simulink model "Simulatie_integral"  (R2018b)
settings: Solver=FixedStepAuto  StartTime=0.0  StopTime=inf  FixedStep=1e-5  RelTol=1e-3
values from neighbouring files (symbols this model uses):
  A = [-(bm*(n^2) + bg)/(Jm*(n^2) + Jg) Kt*n/(Jm*(n^2) + Jg) ... (first row only)    [DC_motor_geared_integral_discrete_sysid23.m]    (also in DC_motor_geared_lqr_discrete_sysid23.m; finalScript.m; finalScriptV2.m; precompensatorVSintegrator.m)
  B = [0 ... (first row only)    [DC_motor_geared_integral_discrete_sysid23.m]    (also in DC_motor_geared_lqr_discrete_sysid23.m; finalScript.m; finalScriptV2.m; precompensatorVSintegrator.m)
  C = [1 0]    [DC_motor_geared_integral_discrete_sysid23.m]    (also in DC_motor_geared_lqr_discrete_sysid23.m = eye(2); finalScript.m; finalScriptV2.m; precompensatorVSintegrator.m = eye(2))
  D = [0]    [DC_motor_geared_integral_discrete_sysid23.m]    (also in DC_motor_geared_lqr_discrete_sysid23.m = [0;0]; finalScript.m; finalScriptV2.m; precompensatorVSintegrator.m)
  Kdi = dlqr(Ad,Bd,Q,R)    [DC_motor_geared_integral_discrete_sysid23.m]    (also in finalScript.m; finalScriptV2.m)
  n = 16.5    [DC_motor_geared_integral_discrete_sysid23.m]    (also in DC_motor_geared_lqr_discrete_sysid23.m; finalScript.m; finalScriptV2.m)
  Tsc = 1/20000    (= 5e-05)    [DC_motor_geared_integral_discrete_sysid23.m]    (also in DC_motor_geared_lqr_discrete_sysid23.m = 1e-05; finalScript.m; finalScriptV2.m = 0.001)
undefined symbols (not defined in the file or in its folder): Add, Bdd, DiscIntNeverNeededParam, sigbuilder_block
libraries: dspswit3 x22, powerlib_meascontrol x17, simulink x11, dspsigops x4, peLuenbergerObserver x2, peGeneralControl x1
settings Model: Creator=BooJC  LastModifiedBy=Roberto
settings SolverCC: AlgebraicLoopSolver=LineSearch
settings DataIOCC: ExternalInput=v_motor_ts
settings DebuggingCC: LibraryContextMissingDiagnostic=none
settings SFSimCC: SimUseLocalCustomCode=off
settings RTWCC: RTWUseLocalCustomCode=off

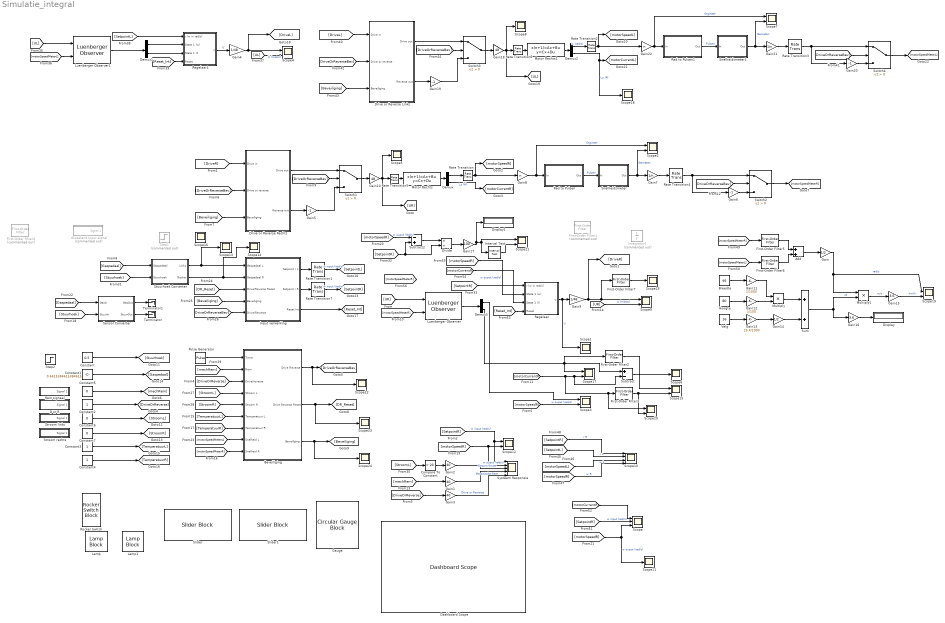
== system Simulatie_integral ==
  Add : Sum
  Beveiliging : Subsystem
  Breedte : Constant  Value=95
  Compare To Constant : simulink/Logic and Bit Operations/Compare To Constant  relop=>  const=20  OutDataTypeStr=boolean
  Constant : Constant  Value=0.5  SampleTime=1/1000
  Constant1 : Constant  Value=0.6615384615384615
  Constant2 : Constant
  Constant3 : Constant
  Constant4 : Constant
  Constant5 : Constant  Value=0
  Constant6 : Constant  Value=0
  Constant7 : Constant  Value=0
  D or R : Subsystem  Tag=STV Subsys  LoadFcn=sigbuilder_block('load');  StartFcn=sigbuilder_block('start');  StopFcn=sigbuilder_block('stop');  ClipboardFcn=sigbuilder_block('clipboard');  mask(Sigbuilder block){tuvar=[0:10]}
      mask help: Simulink:masks:SigbuilderBlock_MD
      mask init:
      | if ~strcmp(get_param(bdroot(gcbh),'SimulationStatus'),'stopped') tuvar = sigbuilder_block('maskInit'); end
      settings: CopyFcn=sigbuilder_block('copy');  DeleteFcn=sigbuilder_block('delete');  ModelCloseFcn=sigbuilder_block('modelClose');  PreSaveFcn=sigbuilder_block('preSave');  PauseFcn=sigbuilder_block('pause');  ContinueFcn=sigbuilder_block('continue');  NameChangeFcn=sigbuilder_block('namechange');  OpenFcn=sigbuilder_block('open',[437.6 153 550.4 359.25 ]);  CloseFcn=sigbuilder_block('close');
      mask Display: plot(0, 0, 100, 100,[2, 2, 32, 32, 2], [68, 8, 8, 68, 68],[32, 2], [38, 38], [32, 19, 2],[53, 60, 44], [32, 17, 17, 2],[16, 16, 31, 31]);txt = getActiveGroup(gcbh);text(2, 100, txt,'verticalAlignment', 'top');
  Dashboard Scope : DashboardScope  WebBlockId=1704  Ymin=-20  Ymax=20
  Demux{,1..3} (4 alike) : Demux  Outputs=2
  Display : Display
  Display1 : Display
  Divide : Product  Inputs=*/
  Drive or Reverse Links : Subsystem
  Drive or Reverse Rechts : Subsystem
  First-Order Filter1 : powerlib_meascontrol/Filters/First-Order Filter  Commented=on  FilterType=Lowpass  Tc=10e-2  Ts=Tsc  Initialize=on  Vac_Init=[0, 0, 50]  Vdc_Init=0  PlotResponse=off  FreqRange="[0,  200,  1]"
      settings: SourceProductName=Simscape Power Systems
  First-Order Filter{2..3,5..7} (5 alike) : powerlib_meascontrol/Filters/First-Order Filter  FilterType=Lowpass  Tc=10e-3  Ts=Tsc  Initialize=on  Vac_Init=[0, 0, 50]  Vdc_Init=0  PlotResponse=off  FreqRange="[0,  200,  1]"
      settings: SourceProductName=Simscape Power Systems
  First-Order Filter4 : powerlib_meascontrol/Filters/First-Order Filter  Commented=on  FilterType=Lowpass  Tc=10e-1  Ts=Tsc  Initialize=on  Vac_Init=[0, 0, 50]  Vdc_Init=0  PlotResponse=off  FreqRange="[0,  200,  1]"
      settings: SourceProductName=Simscape Power Systems
  Gain : Gain  Gain=1/2
  Gain1 : Gain  Gain=40
  Gain10 : Gain  Gain=48
  Gain11 : Gain  Gain=1/1000
  Gain12 : Gain  Gain=1/100
  Gain13 : Gain  Gain=25.4/1000
  Gain14 : Gain  Gain=1/2
  Gain15 : Gain  Gain=3.6
  Gain16 : Gain  Gain=3.6
  Gain17 : Gain  Gain=100
  Gain18 : Gain  Gain=48
  Gain{5..6,19..20} (4 alike) : Gain  Gain=-1
  Gain2 : Gain  Gain=40
  Gain21 : Gain  Gain=1/n
  Gain22 : Gain  Gain=n
  Gain3 : Gain  Gain=40
  Gain4 : Gain  Gain=1/48
  Gain7 : Gain  Gain=1/n
  Gain8 : Gain  Gain=n
  Gain9 : Gain  Gain=1/48
  Gauge : CircularGaugeBlock  WebBlockId=1560  ScaleMin=-50  ScaleMax=50
  Hoogte : Constant  Value=80
  Input verwerking : Subsystem
  Integrator1 : Integrator  Commented=on
  Interval Test : simulink/Logic and Bit Operations/Interval Test  IntervalClosedRight=on  uplimit=2  IntervalClosedLeft=on  lowlimit=-2  OutDataTypeStr=boolean
  Lamp : LampBlock  WebBlockId=1564
  Lamp1 : LampBlock  WebBlockId=1565
  Luenberger Observer : peLuenbergerObserver/Luenberger Observer  StateSpaceType=Discrete-time  Ad=Add  Bd=Bdd  Cd=[1 0]  Dd=0  A=A  B=B  C=C  D=D  ObserverDesign=Observer gain  Ld=L  DesiredEigenvalues=eigenVal  x0=[0 0]  Tsd=0.1  Ts=Tsc
  Luenberger Observer1 : peLuenbergerObserver/Luenberger Observer  StateSpaceType=Discrete-time  Ad=Add  Bd=Bdd  Cd=[1 0]  Dd=0  A=A  B=B  C=C  D=D  ObserverDesign=Observer gain  Ld=L  DesiredEigenvalues=eigenVal  x0=[0 0]  Tsd=0.1  Ts=Tsc
  Motor Rechts : DiscreteStateSpace  A=Add  B=Bdd  C=eye(2)  D=[0; 0]  SampleTime=Tsc
  Motor Rechts1 : DiscreteStateSpace  A=Add  B=Bdd  C=eye(2)  D=[0; 0]  SampleTime=Tsc
  Multiply : Product
  Multiply1 : Product
  Pulse Generator : DiscretePulseGenerator  SampleTime=1/2000
  Rad to Pulsen : Subsystem
  Rad to Pulsen1 : Subsystem
  Rate Transition : RateTransition  OutPortSampleTime=1/100000
  Rate Transition{1,3..7} (6 alike) : RateTransition  OutPortSampleTime=Tsc
  Rate Transition2 : RateTransition  OutPortSampleTime=1/100000
  Regelaar : Subsystem
  Regelaar1 : Subsystem
  Rem signaal : Subsystem  Tag=STV Subsys  LoadFcn=sigbuilder_block('load');  StartFcn=sigbuilder_block('start');  StopFcn=sigbuilder_block('stop');  ClipboardFcn=sigbuilder_block('clipboard');  mask(Sigbuilder block){tuvar=[0:10]}
      mask help: Simulink:masks:SigbuilderBlock_MD
      mask init:
      | if ~strcmp(get_param(bdroot(gcbh),'SimulationStatus'),'stopped') tuvar = sigbuilder_block('maskInit'); end
      settings: CopyFcn=sigbuilder_block('copy');  DeleteFcn=sigbuilder_block('delete');  ModelCloseFcn=sigbuilder_block('modelClose');  PreSaveFcn=sigbuilder_block('preSave');  PauseFcn=sigbuilder_block('pause');  ContinueFcn=sigbuilder_block('continue');  NameChangeFcn=sigbuilder_block('namechange');  OpenFcn=sigbuilder_block('open',[437.6 153 550.4 359.25 ]);  CloseFcn=sigbuilder_block('close');
      mask Display: plot(0, 0, 100, 100,[2, 2, 32, 32, 2], [68, 8, 8, 68, 68],[32, 2], [38, 38], [32, 19, 2],[53, 60, 44], [32, 17, 17, 2],[16, 16, 31, 31]);txt = getActiveGroup(gcbh);text(2, 100, txt,'verticalAlignment', 'top');
  Rocker Switch : RockerSwitchBlock  WebBlockId=1563
      settings: Values={{'Off', 'On'}, [0 1]}
  Scope : Scope  NumInputPorts=3
  Scope{1,5..6,8,11,13..14,16,18,22..25} (13 alike) : Scope
  Scope10 : Scope  NumInputPorts=4
  Scope{2..4,7,9,12,15,17,19..21} (11 alike) : Scope  NumInputPorts=2
  Sensor Converter : Subsystem
  Slider : SliderBlock  WebBlockId=1558  ScaleMax=1
  Slider1 : SliderBlock  WebBlockId=1559  ScaleMax=1
  Snelheidsmeter : Subsystem
  Snelheidsmeter1 : Subsystem
  Step1 : Step  Commented=on  After=3.3  SampleTime=1/100000
  Step2 : Step  Time=0.1  SampleTime=0
  Stroom links : Subsystem  Tag=STV Subsys  LoadFcn=sigbuilder_block('load');  StartFcn=sigbuilder_block('start');  StopFcn=sigbuilder_block('stop');  ClipboardFcn=sigbuilder_block('clipboard');  mask(Sigbuilder block){tuvar=[0:10]}
      mask help: Simulink:masks:SigbuilderBlock_MD
      mask init:
      | if ~strcmp(get_param(bdroot(gcbh),'SimulationStatus'),'stopped') tuvar = sigbuilder_block('maskInit'); end
      settings: CopyFcn=sigbuilder_block('copy');  DeleteFcn=sigbuilder_block('delete');  ModelCloseFcn=sigbuilder_block('modelClose');  PreSaveFcn=sigbuilder_block('preSave');  PauseFcn=sigbuilder_block('pause');  ContinueFcn=sigbuilder_block('continue');  NameChangeFcn=sigbuilder_block('namechange');  OpenFcn=sigbuilder_block('open',[437.6 153 550.4 359.25 ]);  CloseFcn=sigbuilder_block('close');
      mask Display: plot(0, 0, 100, 100,[2, 2, 32, 32, 2], [68, 8, 8, 68, 68],[32, 2], [38, 38], [32, 19, 2],[53, 60, 44], [32, 17, 17, 2],[16, 16, 31, 31]);txt = getActiveGroup(gcbh);text(2, 100, txt,'verticalAlignment', 'top');
  Stroom rechts : Subsystem  Tag=STV Subsys  LoadFcn=sigbuilder_block('load');  StartFcn=sigbuilder_block('start');  StopFcn=sigbuilder_block('stop');  ClipboardFcn=sigbuilder_block('clipboard');  mask(Sigbuilder block){tuvar=[0:10]}
      mask help: Simulink:masks:SigbuilderBlock_MD
      mask init:
      | if ~strcmp(get_param(bdroot(gcbh),'SimulationStatus'),'stopped') tuvar = sigbuilder_block('maskInit'); end
      settings: CopyFcn=sigbuilder_block('copy');  DeleteFcn=sigbuilder_block('delete');  ModelCloseFcn=sigbuilder_block('modelClose');  PreSaveFcn=sigbuilder_block('preSave');  PauseFcn=sigbuilder_block('pause');  ContinueFcn=sigbuilder_block('continue');  NameChangeFcn=sigbuilder_block('namechange');  OpenFcn=sigbuilder_block('open',[437.6 153 550.4 359.25 ]);  CloseFcn=sigbuilder_block('close');
      mask Display: plot(0, 0, 100, 100,[2, 2, 32, 32, 2], [68, 8, 8, 68, 68],[32, 2], [38, 38], [32, 19, 2],[53, 60, 44], [32, 17, 17, 2],[16, 16, 31, 31]);txt = getActiveGroup(gcbh);text(2, 100, txt,'verticalAlignment', 'top');
  Stuurhoek Converter : Subsystem
  Subtract : Sum  Inputs=+-
  Subtract2 : Sum  Inputs=-+
  Sum : Sum
  Switch{1..4} (4 alike) : Switch  Criteria=u2 > Threshold
  Systeem Responsie : Scope  NumInputPorts=5
  Terminator : Terminator
  Terminator1 : Terminator
  Velg : Constant  Value=16
  Wisselend Input signal : Subsystem  Tag=STV Subsys  Commented=on  LoadFcn=sigbuilder_block('load');  StartFcn=sigbuilder_block('start');  StopFcn=sigbuilder_block('stop');  ClipboardFcn=sigbuilder_block('clipboard');  mask(Sigbuilder block){tuvar=[0:10]}
      mask help: Simulink:masks:SigbuilderBlock_MD
      mask init:
      | if ~strcmp(get_param(bdroot(gcbh),'SimulationStatus'),'stopped') tuvar = sigbuilder_block('maskInit'); end
      settings: CopyFcn=sigbuilder_block('copy');  DeleteFcn=sigbuilder_block('delete');  ModelCloseFcn=sigbuilder_block('modelClose');  PreSaveFcn=sigbuilder_block('preSave');  PauseFcn=sigbuilder_block('pause');  ContinueFcn=sigbuilder_block('continue');  NameChangeFcn=sigbuilder_block('namechange');  OpenFcn=sigbuilder_block('open',[437.6 153 550.4 359.25 ]);  CloseFcn=sigbuilder_block('close');
      mask Display: plot(0, 0, 100, 100,[2, 2, 32, 32, 2], [68, 8, 8, 68, 68],[32, 2], [38, 38], [32, 19, 2],[53, 60, 44], [32, 17, 17, 2],[16, 16, 31, 31]);txt = getActiveGroup(gcbh);text(2, 100, txt,'verticalAlignment', 'top');
  wires:
  Rate Transition1/1 -> [SetpointL]  "w input (rad/s)"
  Demux/2 -> [motorCurrentR]  "I_s (A)"
  Constant5/1 -> [mechRem]
  [DriveR] -> Drive or Reverse Rechts/1(Drive in)
  [DriveOrReverseBev] -> Drive or Reverse Rechts/2(Drive or reverse)
  Demux3/2 -> First-Order Filter2/1, Scope17/1, Subtract/1
  [motorCurrentR] -> Scope20/1, First-Order Filter3/1, Subtract/2, Scope17/2
  [motorSpeedR] -> Scope3/2  "w ouput (rad/s)"
  Demux3/1 -> Scope3/1
  Rad to Pulsen/1(Out) -> Snelheidsmeter/1(In)  "Pulsen"
  [motorSpeedMeterR] -> Luenberger Observer/2
  Snelheidsmeter/1(Out) -> Gain7/1, Scope2/2  "Gemeten"
  Gain8/1 -> Rad to Pulsen/1(In), Scope2/1  "Orgineel"
  Gain7/1 -> Rate Transition4/1
  Gain10/1 -> Rate Transition5/1, Scope5/1, [UR]
  [UR] -> Luenberger Observer/1
  Subtract/1 -> Scope6/1
  Rate Transition/1 -> [motorSpeedR], Gain8/1
  Regelaar/1(u) -> Scope1/1, Gain9/1  "U"
  Rate Transition5/1 -> Motor Rechts/1
  [UR] -> Scope9/2  "U (motor)"
  Pulse Generator/1 -> Beveiliging/1(Timer)
  Drive or Reverse Rechts/1(Drive out) -> Switch1/1
  Drive or Reverse Rechts/2(Reverse out) -> Gain5/1
  Switch1/1 -> Gain10/1
  [DriveOrReverseBev] -> Switch1/2
  Gain5/1 -> Switch1/3
  Gain6/1 -> Switch2/3
  Rate Transition4/1 -> Gain6/1, Switch2/1
  Switch2/1 -> [motorSpeedMeterR]
  First-Order Filter2/1 -> Scope15/1
  First-Order Filter3/1 -> Scope20/2, Scope15/2
  Gain9/1 -> [DriveR], First-Order Filter7/1, Scope9/1
  [Gaspedaal] -> Stuurhoek Converter/1("Gaspedaal ")
  [Beveiliging] -> Drive or Reverse Rechts/3(Beveiliging)
  Hoogte/1 -> Gain12/1
  Gain11/1 -> Multiply/1
  Gain13/1 -> Gain14/1
  Breedte/1 -> Gain11/1
  Gain14/1 -> Sum/2
  Multiply/1 -> Sum/1
  Gain12/1 -> Multiply/2
  Velg/1 -> Gain13/1
  Gain/1 -> Multiply1/1, Scope19/1  "rad/s"
  Sum/1 -> Gain16/1, Multiply1/2  "r0"
  Multiply1/1 -> Gain15/1  "m/s"
  Gain15/1 -> Scope19/2  "km/h"
  Gain16/1 -> Display/1
  Input verwerking/1(Setpoint r L) -> Rate Transition1/1
  [Stuurhoek] -> Stuurhoek Converter/2(Stuurhoek)
  [motorSpeedR] -> Subtract2/1  "w ouput (rad/s)"
  Subtract2/1 -> Divide/1
  Gain17/1 -> Display1/1, Interval Test/1, Scope21/1
  Divide/1 -> Gain17/1
  [motorSpeedMeterL] -> Beveiliging/8(Snelheid L)
  [motorSpeedMeterR] -> Beveiliging/9(Snelheid R)
  [StroomL] -> Beveiliging/4(Stroom L)
  [DR_Reset] -> Input verwerking/3(Drive/Reverse Reset)
  Beveiliging/3(Beveiliging) -> Scope24/1, [Beveiliging]
  [Beveiliging] -> Input verwerking/4(Beveiliging)
  [DriveOrReverse] -> Beveiliging/3(Drive/reverse)
  Beveiliging/1("Drive Reverse ") -> Scope22/1, [DriveOrReverseBev]
  [DriveOrReverseBev] -> Input verwerking/5(Drive/Reverse)
  [DriveOrReverseBev] -> Switch2/2
  Gain3/1 -> Systeem Responsie/5  "Drive or Reverse"
  [mechRem] -> Gain1/1
  Compare To Constant/1 -> Gain2/1
  Gain2/1 -> Systeem Responsie/3  "Stroom limiet"
  [DriveOrReverse] -> Gain3/1
  [motorSpeedR] -> Scope12/2, Systeem Responsie/2  "w ouput (rad/s)"
  [SetpointR] -> Scope12/1, Systeem Responsie/1  "w input (rad/s)"
  Gain1/1 -> Systeem Responsie/4  "Mecanische Rem"
  [StroomL] -> Compare To Constant/1
  Luenberger Observer/1 -> Demux3/1
  Constant2/1 -> [DriveOrReverse]
  Constant6/1 -> [StroomL]
  Constant7/1 -> [StroomR]
  Constant/1 -> [Stuurhoek]
  Constant1/1 -> [Gaspedaal]
  Constant3/1 -> [TemperatuurL]
  Constant4/1 -> [TemperatuurR]
  [TemperatuurL] -> Beveiliging/6(Temperatuur L)
  [TemperatuurR] -> Beveiliging/7(Temperatuur R)
  [StroomR] -> Beveiliging/5(Stroom R)
  [mechRem] -> Beveiliging/2(Rem)
  [Stuurhoek] -> Sensor Converter/2(StuurIn)
  [Gaspedaal] -> Sensor Converter/1(GasIn)
  Sensor Converter/2(StuurOut) -> Terminator/1
  Sensor Converter/1(GasOut) -> Terminator1/1
  Input verwerking/3(Reset Int) -> [Reset_Int]
  [SetpointR] -> Divide/2, Subtract2/2
  [SetpointR] -> Regelaar/1(r (w in rad/s))
  [Reset_Int] -> Regelaar/4(Reset)
  [UL] -> Scope4/2  "U (motor)"
  [motorSpeedMeterL] -> Luenberger Observer1/2
  [UL] -> Luenberger Observer1/1
  Gain4/1 -> [DriveL], Scope4/1
  Regelaar1/1(u) -> Gain4/1  "U"
  Luenberger Observer1/1 -> Demux1/1
  [Reset_Int] -> Regelaar1/4(Reset)
  [SetpointL] -> Regelaar1/1(r (w in rad/s))
  Drive or Reverse Links/2(Reverse out) -> Gain19/1
  Switch3/1 -> Gain18/1
  [DriveL] -> Drive or Reverse Links/1(Drive in)
  Switch4/1 -> [motorSpeedMeterL]
  Gain20/1 -> Switch4/3
  Gain22/1 -> Rad to Pulsen1/1(In), Scope7/1  "Orgineel"
  Drive or Reverse Links/1(Drive out) -> Switch3/1
  [Beveiliging] -> Drive or Reverse Links/3(Beveiliging)
  Gain19/1 -> Switch3/3
  Demux2/1 -> Rate Transition2/1  "w (rad/s)"
  Gain18/1 -> Rate Transition6/1, Scope8/1, [UL]
  Rate Transition2/1 -> [motorSpeedL], Gain22/1
  Rate Transition3/1 -> Gain20/1, Switch4/1
  Motor Rechts1/1 -> Demux2/1
  Gain21/1 -> Rate Transition3/1
  Rate Transition6/1 -> Motor Rechts1/1
  Snelheidsmeter1/1(Out) -> Gain21/1, Scope7/2  "Gemeten"
  [DriveOrReverseBev] -> Drive or Reverse Links/2(Drive or reverse)
  [DriveOrReverseBev] -> Switch3/2
  Demux2/2 -> Scope18/1, [motorCurrentL]  "I_s (A)"
  Rad to Pulsen1/1(Out) -> Snelheidsmeter1/1(In)  "Pulsen"
  [DriveOrReverseBev] -> Switch4/2
  [SetpointL] -> Scope10/2  "r L"
  [motorSpeedL] -> Scope10/3  "w L"
  [motorSpeedR] -> Scope10/4  "w R"
  Stuurhoek Converter/1(Links) -> Scope13/1, Input verwerking/1(Gaspedaal L)
  Stuurhoek Converter/2(Rechts) -> Scope14/1, Input verwerking/2(Gaspedaal R)
  Rate Transition7/1 -> [SetpointR]  "w input (rad/s)"
  Input verwerking/2(Setpoint r R) -> Rate Transition7/1
  [SetpointR] -> Scope10/1  "r R"
  [motorSpeedMeterR] -> First-Order Filter5/1
  First-Order Filter5/1 -> Add/1
  First-Order Filter6/1 -> Add/2
  [motorSpeedMeterL] -> First-Order Filter6/1
  Add/1 -> Gain/1
  [motorSpeedR] -> Scope11/1, Scope/3  "w ouput (rad/s)"
  [SetpointR] -> Scope/2  "w input (rad/s)"
  [motorCurrentR] -> Scope/1
  Interval Test/1 -> Scope21/2
  Beveiliging/2(Drive Reverse Reset) -> Scope23/1, [DR_Reset]
  Motor Rechts/1 -> Demux/1
  Demux/1 -> Rate Transition/1
  Demux1/1 -> Regelaar1/2(State 1 (w))
  Demux1/2 -> Regelaar1/3(State 1 (I))
  First-Order Filter7/1 -> Scope25/1
  [motorSpeedR] -> Regelaar/2(State 1 (w))  "w ouput (rad/s)"
  [motorCurrentR] -> Regelaar/3(State 1 (I))

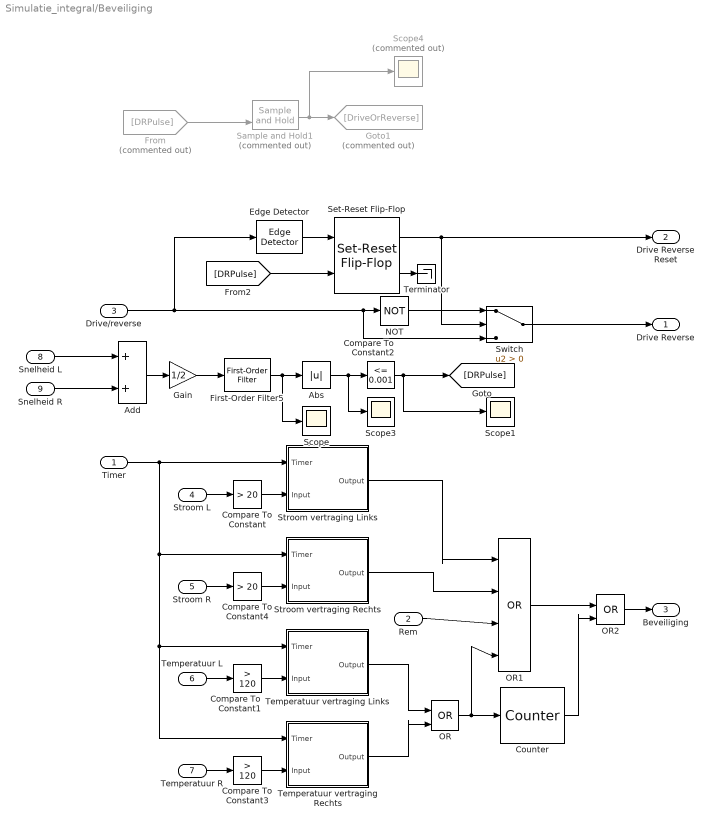
== system Simulatie_integral/Beveiliging ==
  Timer : Inport
  Rem : Inport  Port=2
  Drive/reverse : Inport  Port=3
  Stroom L : Inport  Port=4
  Stroom R : Inport  Port=5
  Temperatuur L : Inport  Port=6
  Temperatuur R : Inport  Port=7
  Snelheid L : Inport  Port=8
  Snelheid R : Inport  Port=9
  Abs : Abs
  Add : Sum
  Compare To Constant : simulink/Logic and Bit Operations/Compare To Constant  relop=>  const=20  OutDataTypeStr=boolean
  Compare To Constant1 : simulink/Logic and Bit Operations/Compare To Constant  relop=>  const=120  OutDataTypeStr=boolean
  Compare To Constant2 : simulink/Logic and Bit Operations/Compare To Constant  relop=<=  const=0.001  OutDataTypeStr=boolean
  Compare To Constant3 : simulink/Logic and Bit Operations/Compare To Constant  relop=>  const=120  OutDataTypeStr=boolean
  Compare To Constant4 : simulink/Logic and Bit Operations/Compare To Constant  relop=>  const=20  OutDataTypeStr=boolean
  Counter : dspswit3/Counter  Direction=Up  CountEvent=Rising edge  CounterSize=32 bits  MaxCount=255  InitialCount=0  Output=Hit  HitValue=3  ResetInput=off  SamplesPerFrame=1  Ts=1  CntDtype=double  HitDtype=Logical
  Edge Detector : powerlib_meascontrol/Logic/Edge Detector  model=Either  ic=0  Ts=-1
      settings: SourceProductName=Simscape Power Systems  SourceProductBaseCode=PS
  First-Order Filter5 : powerlib_meascontrol/Filters/First-Order Filter  FilterType=Lowpass  Tc=10e-3  Ts=Tsc  Initialize=on  Vac_Init=[0, 0, 50]  Vdc_Init=0  PlotResponse=off  FreqRange="[0,  200,  1]"
      settings: SourceProductName=Simscape Power Systems
  From : From  Commented=on  GotoTag=DRPulse
  Gain : Gain  Gain=1/2
  Goto1 : Goto  Commented=on  GotoTag=DriveOrReverse
  NOT : Logic  Operator=NOT  IconShape=distinctive  AllPortsSameDT=off  OutDataTypeStr=boolean
  OR : Logic  Operator=OR  IconShape=distinctive  AllPortsSameDT=off  OutDataTypeStr=boolean
  OR1 : Logic  Operator=OR  Inputs=4  IconShape=distinctive  AllPortsSameDT=off  OutDataTypeStr=boolean
  OR2 : Logic  Operator=OR  IconShape=distinctive  AllPortsSameDT=off  OutDataTypeStr=boolean
  Sample and Hold1 : powerlib_meascontrol/Additional Components/Sample and Hold  Commented=on  ic=0  Ts=0
      settings: SourceProductName=Simscape Power Systems  SourceProductBaseCode=PS
  Scope : Scope
  Scope1 : Scope
  Scope3 : Scope
  Scope4 : Scope  Commented=on
  Set-Reset Flip-Flop : peGeneralControl/Set-Reset Flip-Flop  LabelModeActiveChoice=Discrete  UndefState=Set  Q0=0  Ts=-1
  Stroom vertraging Links : Subsystem
  Stroom vertraging Rechts : Subsystem
  Switch : Switch  Criteria=u2 > Threshold
  Temperatuur vertraging Links : Subsystem
  "Temperatuur vertraging Rechts " : Subsystem
  Terminator : Terminator
  "Drive Reverse " : Outport
  Drive Reverse Reset : Outport  Port=2
  Beveiliging : Outport  Port=3
  wires:
  Compare To Constant/1 -> Stroom vertraging Links/2(Input)
  Stroom L/1 -> Compare To Constant/1
  Compare To Constant1/1 -> Temperatuur vertraging Links/2(Input)
  Temperatuur L/1 -> Compare To Constant1/1
  Edge Detector/1 -> Set-Reset Flip-Flop/1
  Set-Reset Flip-Flop/1 -> Switch/2, Drive Reverse Reset/1
  Sample and Hold1/1 -> Scope4/1, Goto1/1
  Abs/1 -> Scope3/1, Compare To Constant2/1
  Compare To Constant2/1 -> [DRPulse], Scope1/1
  [DRPulse] -> Set-Reset Flip-Flop/2
  Drive/reverse/1 -> Edge Detector/1, Switch/3, NOT/1
  From/1 -> Sample and Hold1/2
  Snelheid L/1 -> Add/1
  Snelheid R/1 -> Add/2
  Add/1 -> Gain/1
  Gain/1 -> First-Order Filter5/1
  Compare To Constant3/1 -> "Temperatuur vertraging Rechts "/2(Input)
  Timer/1 -> Stroom vertraging Links/1(Timer), Stroom vertraging Rechts/1(Timer), "Temperatuur vertraging Rechts "/1(Timer), Temperatuur vertraging Links/1(Timer)
  Compare To Constant4/1 -> Stroom vertraging Rechts/2(Input)
  Stroom R/1 -> Compare To Constant4/1
  Rem/1 -> OR1/3
  Stroom vertraging Links/1(Output) -> OR1/1
  Stroom vertraging Rechts/1(Output) -> OR1/2
  Switch/1 -> "Drive Reverse "/1
  NOT/1 -> Switch/1
  OR/1 -> OR1/4, Counter/1
  Temperatuur vertraging Links/1(Output) -> OR/1
  "Temperatuur vertraging Rechts "/1(Output) -> OR/2
  OR2/1 -> Beveiliging/1
  Counter/1 -> OR2/2
  OR1/1 -> OR2/1
  Temperatuur R/1 -> Compare To Constant3/1
  Set-Reset Flip-Flop/2 -> Terminator/1
  First-Order Filter5/1 -> Scope/1, Abs/1

== system Simulatie_integral/D or R ==
  Demux : Demux  Tag=STV Demux  Outputs=1
  FromWs : FromWorkspace  Tag=STV FromWs  VariableName=tuvar  SampleTime=0
      SigBuilderData=|
      | common.afterFinalStr = 'Extrapolate'
      | common.sampleTime = 0
      | dataSet.timeRange = [0 10]
      | dataSet.name = 'Group 1'
      | sbobj.Groups.Name = 'Group 1'
      | sbobj.Groups.Signals.Name = 'Signal 1'
      | sbobj.Groups.Signals.XData = [0 2 2 4 4 6.5 6.5 9.6 9.6 10]
      | sbobj.Groups.Signals.YData = [0 0 1 1 0 0 1 1 0 0]
  Signal 1 : Outport  Tag=STV Outport
  wires:
  Demux/1 -> Signal 1/1
  FromWs/1 -> Demux/1

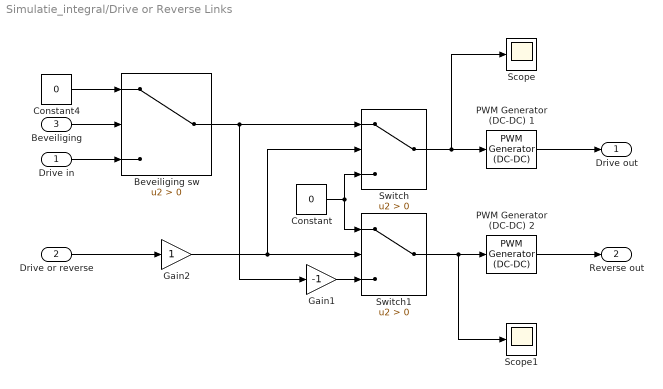
== system Simulatie_integral/Drive or Reverse Links ==
  Drive in : Inport
  Drive or reverse : Inport  Port=2
  Beveiliging : Inport  Port=3
  Beveiliging sw : Switch  Criteria=u2 > Threshold
  Constant : Constant  Value=0
  Constant4 : Constant  Value=0
  Gain1 : Gain  Gain=-1
  Gain2 : Gain
  PWM Generator (DC-DC) 1 : powerlib_meascontrol/Pulse & Signal Generators/PWM Generator (DC-DC)  Fsw=20e3  Ts=1/100000
      settings: SourceProductName=Simscape Electrical
  PWM Generator (DC-DC) 2 : powerlib_meascontrol/Pulse & Signal Generators/PWM Generator (DC-DC)  Fsw=20e3  Ts=1/100000
      settings: SourceProductName=Simscape Electrical
  Scope : Scope
  Scope1 : Scope
  Switch : Switch  Criteria=u2 > Threshold
  Switch1 : Switch  Criteria=u2 > Threshold
  Drive out : Outport
  Reverse out : Outport  Port=2
  wires:
  Gain1/1 -> Switch1/3
  Switch1/1 -> Scope1/1, PWM Generator (DC-DC) 2/1
  Switch/1 -> Scope/1, PWM Generator (DC-DC) 1/1
  Constant4/1 -> Beveiliging sw/1
  Constant/1 -> Switch1/1, Switch/3
  Beveiliging sw/1 -> Gain1/1, Switch/1
  Drive in/1 -> Beveiliging sw/3
  Beveiliging/1 -> Beveiliging sw/2
  PWM Generator (DC-DC) 1/1 -> Drive out/1
  PWM Generator (DC-DC) 2/1 -> Reverse out/1
  Gain2/1 -> Switch/2, Switch1/2
  Drive or reverse/1 -> Gain2/1

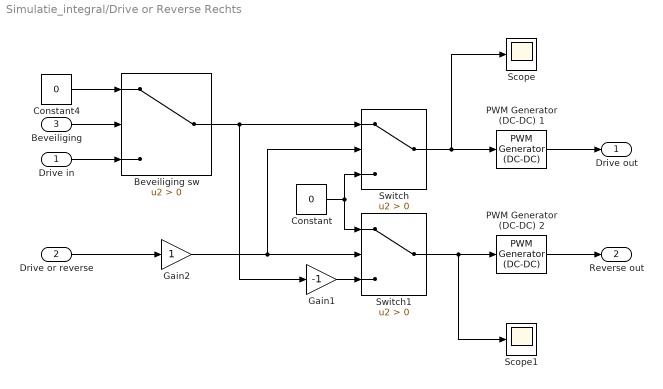
== system Simulatie_integral/Drive or Reverse Rechts ==
  Drive in : Inport
  Drive or reverse : Inport  Port=2
  Beveiliging : Inport  Port=3
  Beveiliging sw : Switch  Criteria=u2 > Threshold
  Constant : Constant  Value=0
  Constant4 : Constant  Value=0
  Gain1 : Gain  Gain=-1
  Gain2 : Gain
  PWM Generator (DC-DC) 1 : powerlib_meascontrol/Pulse & Signal Generators/PWM Generator (DC-DC)  Fsw=20e3  Ts=1/100000
      settings: SourceProductName=Simscape Electrical
  PWM Generator (DC-DC) 2 : powerlib_meascontrol/Pulse & Signal Generators/PWM Generator (DC-DC)  Fsw=20e3  Ts=1/100000
      settings: SourceProductName=Simscape Electrical
  Scope : Scope
  Scope1 : Scope
  Switch : Switch  Criteria=u2 > Threshold
  Switch1 : Switch  Criteria=u2 > Threshold
  Drive out : Outport
  Reverse out : Outport  Port=2
  wires:
  Gain1/1 -> Switch1/3
  Switch1/1 -> Scope1/1, PWM Generator (DC-DC) 2/1
  Constant4/1 -> Beveiliging sw/1
  Constant/1 -> Switch1/1, Switch/3
  Beveiliging sw/1 -> Gain1/1, Switch/1
  Drive in/1 -> Beveiliging sw/3
  Beveiliging/1 -> Beveiliging sw/2
  Switch/1 -> PWM Generator (DC-DC) 1/1, Scope/1
  PWM Generator (DC-DC) 2/1 -> Reverse out/1
  Gain2/1 -> Switch/2, Switch1/2
  Drive or reverse/1 -> Gain2/1
  PWM Generator (DC-DC) 1/1 -> Drive out/1

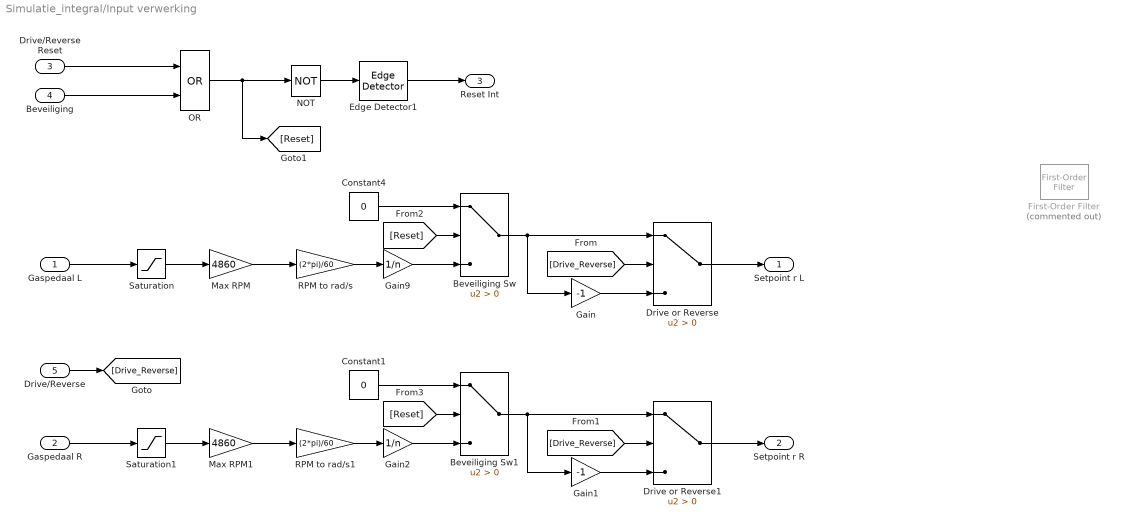
== system Simulatie_integral/Input verwerking ==
  Gaspedaal L : Inport
  Gaspedaal R : Inport  Port=2
  Drive/Reverse Reset : Inport  Port=3
  Beveiliging : Inport  Port=4
  Drive/Reverse : Inport  Port=5
  Beveiliging Sw : Switch  Criteria=u2 > Threshold
  Beveiliging Sw1 : Switch  Criteria=u2 > Threshold
  Constant1 : Constant  Value=0
  Constant4 : Constant  Value=0
  Drive or Reverse : Switch  Criteria=u2 > Threshold
  Drive or Reverse1 : Switch  Criteria=u2 > Threshold
  Edge Detector1 : dspswit3/Edge Detector  InputProcessing=Columns as channels (frame based)
      settings: SourceProductName=DSP System Toolbox  SourceProductBaseCode=DS
  First-Order Filter : powerlib_meascontrol/Filters/First-Order Filter  Commented=on  FilterType=Lowpass  Tc=10e-2  Ts=0  Initialize=on  Vac_Init=[0, 0, 60]  Vdc_Init=0  PlotResponse=off  FreqRange="[0,  200,  1]"
      settings: SourceProductName=Simscape Power Systems
  Gain : Gain  Gain=-1
  Gain1 : Gain  Gain=-1
  Gain2 : Gain  Gain=1/n
  Gain9 : Gain  Gain=1/n
  Max RPM : Gain  Gain=4860
  Max RPM1 : Gain  Gain=4860
  NOT : Logic  Operator=NOT  IconShape=distinctive  AllPortsSameDT=off  OutDataTypeStr=boolean
  OR : Logic  Operator=OR  IconShape=distinctive  AllPortsSameDT=off  OutDataTypeStr=boolean
  RPM to rad/s : Gain  Gain=(2*pi)/60
  RPM to rad/s1 : Gain  Gain=(2*pi)/60
  Saturation : Saturate  UpperLimit=inf  LowerLimit=0
  Saturation1 : Saturate  UpperLimit=inf  LowerLimit=0
  Setpoint r L : Outport
  Setpoint r R : Outport  Port=2
  Reset Int : Outport  Port=3
  wires:
  Constant4/1 -> Beveiliging Sw/1
  Max RPM/1 -> RPM to rad/s/1
  Saturation/1 -> Max RPM/1
  RPM to rad/s/1 -> Gain9/1
  Gaspedaal L/1 -> Saturation/1
  OR/1 -> [Reset], NOT/1
  Gain9/1 -> Beveiliging Sw/3
  Beveiliging Sw/1 -> Gain/1, Drive or Reverse/1
  Gain/1 -> Drive or Reverse/3
  [Drive_Reverse] -> Drive or Reverse/2
  Drive or Reverse/1 -> Setpoint r L/1
  Edge Detector1/1 -> Reset Int/1
  NOT/1 -> Edge Detector1/1
  Beveiliging/1 -> OR/2
  Drive/Reverse Reset/1 -> OR/1
  Max RPM1/1 -> RPM to rad/s1/1
  Saturation1/1 -> Max RPM1/1
  RPM to rad/s1/1 -> Gain2/1
  Drive or Reverse1/1 -> Setpoint r R/1
  Gaspedaal R/1 -> Saturation1/1
  Gain1/1 -> Drive or Reverse1/3
  Beveiliging Sw1/1 -> Gain1/1, Drive or Reverse1/1
  Constant1/1 -> Beveiliging Sw1/1
  [Drive_Reverse] -> Drive or Reverse1/2
  Gain2/1 -> Beveiliging Sw1/3
  Drive/Reverse/1 -> [Drive_Reverse]
  [Reset] -> Beveiliging Sw/2
  [Reset] -> Beveiliging Sw1/2

== system Simulatie_integral/Rad to Pulsen ==
  In : Inport
  Abs : Abs
  Compare To Constant1 : simulink/Logic and Bit Operations/Compare To Constant  relop=<=  const=0.5  OutDataTypeStr=boolean
  Discrete-Time Integrator : DiscreteIntegrator  SampleTime=-1  ICPrevOutput=DiscIntNeverNeededParam  ICPrevScaledInput=DiscIntNeverNeededParam
  Gain : Gain  Gain=500/(2*pi)
  Rounding Function : Rounding
  Sum1 : Sum  Inputs=|+-
  Out : Outport
  wires:
  Rounding Function/1 -> Sum1/2
  Discrete-Time Integrator/1 -> Rounding Function/1, Sum1/1
  Compare To Constant1/1 -> Out/1
  Sum1/1 -> Compare To Constant1/1
  Gain/1 -> Discrete-Time Integrator/1
  In/1 -> Abs/1
  Abs/1 -> Gain/1

== system Simulatie_integral/Rad to Pulsen1 ==
  In : Inport
  Abs2 : Abs
  Compare To Constant1 : simulink/Logic and Bit Operations/Compare To Constant  relop=<=  const=0.5  OutDataTypeStr=boolean
  Discrete-Time Integrator : DiscreteIntegrator  SampleTime=-1  ICPrevOutput=DiscIntNeverNeededParam  ICPrevScaledInput=DiscIntNeverNeededParam
  Gain : Gain  Gain=500/(2*pi)
  Rounding Function : Rounding
  Sum1 : Sum  Inputs=|+-
  Out : Outport
  wires:
  Rounding Function/1 -> Sum1/2
  Discrete-Time Integrator/1 -> Rounding Function/1, Sum1/1
  Compare To Constant1/1 -> Out/1
  Sum1/1 -> Compare To Constant1/1
  Gain/1 -> Discrete-Time Integrator/1
  In/1 -> Abs2/1
  Abs2/1 -> Gain/1

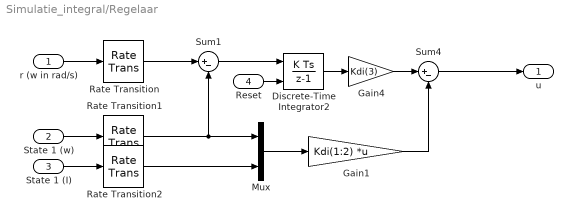
== system Simulatie_integral/Regelaar ==
  r (w in rad/s) : Inport
  State 1 (w) : Inport  Port=2
  State 1 (I) : Inport  Port=3
  Reset : Inport  Port=4
  Discrete-Time Integrator2 : DiscreteIntegrator  gainval=1  ExternalReset=rising  SampleTime=Tsc  ICPrevOutput=DiscIntNeverNeededParam  ICPrevScaledInput=DiscIntNeverNeededParam
  Gain1 : Gain  Gain=Kdi(1:2)  Multiplication=Matrix(K*u)
  Gain4 : Gain  Gain=Kdi(3)
  Mux : Mux  Inputs=2
  Rate Transition : RateTransition  OutPortSampleTime=Tsc
  Rate Transition1 : RateTransition  OutPortSampleTime=Tsc
  Rate Transition2 : RateTransition  OutPortSampleTime=Tsc
  Sum1 : Sum  Inputs=|+-
  Sum4 : Sum  Inputs=|+-
  u : Outport
  wires:
  r (w in rad/s)/1 -> Rate Transition/1
  State 1 (I)/1 -> Rate Transition2/1
  Mux/1 -> Gain1/1
  Gain1/1 -> Sum4/2
  Gain4/1 -> Sum4/1
  Sum4/1 -> u/1
  State 1 (w)/1 -> Rate Transition1/1
  Sum1/1 -> Discrete-Time Integrator2/1
  Discrete-Time Integrator2/1 -> Gain4/1
  Reset/1 -> Discrete-Time Integrator2/2
  Rate Transition/1 -> Sum1/1
  Rate Transition1/1 -> Mux/1, Sum1/2
  Rate Transition2/1 -> Mux/2

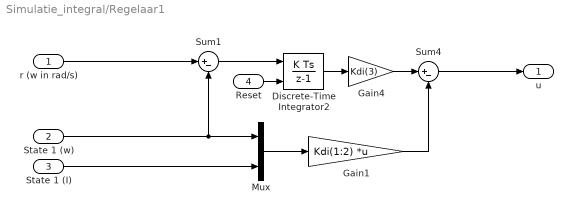
== system Simulatie_integral/Regelaar1 ==
  r (w in rad/s) : Inport
  State 1 (w) : Inport  Port=2
  State 1 (I) : Inport  Port=3
  Reset : Inport  Port=4
  Discrete-Time Integrator2 : DiscreteIntegrator  gainval=1  ExternalReset=rising  SampleTime=Tsc  ICPrevOutput=DiscIntNeverNeededParam  ICPrevScaledInput=DiscIntNeverNeededParam
  Gain1 : Gain  Gain=Kdi(1:2)  Multiplication=Matrix(K*u)
  Gain4 : Gain  Gain=Kdi(3)
  Mux : Mux  Inputs=2
  Sum1 : Sum  Inputs=|+-
  Sum4 : Sum  Inputs=|+-
  u : Outport
  wires:
  r (w in rad/s)/1 -> Sum1/1
  State 1 (I)/1 -> Mux/2
  Mux/1 -> Gain1/1
  Gain1/1 -> Sum4/2
  Gain4/1 -> Sum4/1
  Sum4/1 -> u/1
  State 1 (w)/1 -> Mux/1, Sum1/2
  Sum1/1 -> Discrete-Time Integrator2/1
  Discrete-Time Integrator2/1 -> Gain4/1
  Reset/1 -> Discrete-Time Integrator2/2

== system Simulatie_integral/Rem signaal ==
  Demux : Demux  Tag=STV Demux  Outputs=1
  FromWs : FromWorkspace  Tag=STV FromWs  VariableName=tuvar  SampleTime=0
      SigBuilderData=|
      | common.afterFinalStr = 'Extrapolate'
      | common.sampleTime = 0
      | dataSet.timeRange = [0 10]
      | dataSet.name = 'Group 1'
      | sbobj.Groups.Name = 'Group 1'
      | sbobj.Groups.Signals.Name = 'Signal 1'
      | sbobj.Groups.Signals.XData = [0 6 6 7 7 9 9 9.6 9.6 10]
      | sbobj.Groups.Signals.YData = [0 0 1 1 0 0 1 1 0 0]
  Signal 1 : Outport  Tag=STV Outport
  wires:
  Demux/1 -> Signal 1/1
  FromWs/1 -> Demux/1

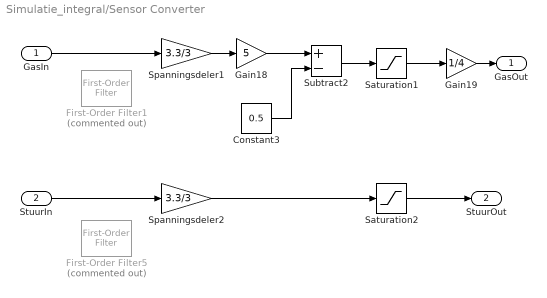
== system Simulatie_integral/Sensor Converter ==
  GasIn : Inport
  StuurIn : Inport  Port=2
  Constant3 : Constant  Value=0.5
  First-Order Filter1 : powerlib_meascontrol/Filters/First-Order Filter  Commented=on  FilterType=Lowpass  Tc=1e-3  Ts=Tsc  Initialize=on  Vac_Init=[0, 0, 50]  Vdc_Init=0  PlotResponse=off  FreqRange="[0,  200,  1]"
      settings: SourceProductName=Simscape Power Systems
  First-Order Filter5 : powerlib_meascontrol/Filters/First-Order Filter  Commented=on  FilterType=Lowpass  Tc=1e-3  Ts=Tsc  Initialize=on  Vac_Init=[0, 0, 50]  Vdc_Init=0  PlotResponse=off  FreqRange="[0,  200,  1]"
      settings: SourceProductName=Simscape Power Systems
  Gain18 : Gain  Gain=5
  Gain19 : Gain  Gain=1/4
  Saturation1 : Saturate  UpperLimit=4  LowerLimit=0
  Saturation2 : Saturate  UpperLimit=1  LowerLimit=0
  Spanningsdeler1 : Gain  Gain=3.3/3
  Spanningsdeler2 : Gain  Gain=3.3/3
  Subtract2 : Sum  Inputs=+-
  GasOut : Outport
  StuurOut : Outport  Port=2
  wires:
  Constant3/1 -> Subtract2/2
  Saturation1/1 -> Gain19/1
  GasIn/1 -> Spanningsdeler1/1
  Spanningsdeler1/1 -> Gain18/1
  Gain18/1 -> Subtract2/1
  Gain19/1 -> GasOut/1
  Subtract2/1 -> Saturation1/1
  Saturation2/1 -> StuurOut/1
  Spanningsdeler2/1 -> Saturation2/1
  StuurIn/1 -> Spanningsdeler2/1

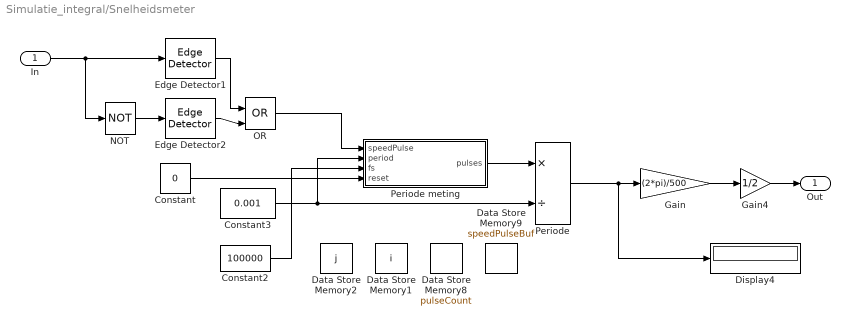
== system Simulatie_integral/Snelheidsmeter ==
  In : Inport
  Constant : Constant  Value=0
  Constant2 : Constant  Value=100000
  Constant3 : Constant  Value=0.001
  Data Store Memory1 : DataStoreMemory  DataStoreName=i  ReadBeforeWriteMsg=warning  WriteAfterWriteMsg=warning  WriteAfterReadMsg=warning  InitialValue=1  ShowAdditionalParam=off  OutDataTypeStr=uint32
  Data Store Memory2 : DataStoreMemory  DataStoreName=j  ReadBeforeWriteMsg=warning  WriteAfterWriteMsg=warning  WriteAfterReadMsg=warning  InitialValue=2  ShowAdditionalParam=off  OutDataTypeStr=uint32
  Data Store Memory8 : DataStoreMemory  DataStoreName=pulseCount  ReadBeforeWriteMsg=warning  WriteAfterWriteMsg=warning  WriteAfterReadMsg=warning  ShowAdditionalParam=off  OutDataTypeStr=uint32
  Data Store Memory9 : DataStoreMemory  DataStoreName=speedPulseBuf  ReadBeforeWriteMsg=warning  WriteAfterWriteMsg=warning  WriteAfterReadMsg=warning  ShowAdditionalParam=off  OutDataTypeStr=uint8  Dimensions=10001
  Display4 : Display
  Edge Detector1 : dspswit3/Edge Detector  InputProcessing=Columns as channels (frame based)
      settings: SourceProductName=DSP System Toolbox  SourceProductBaseCode=DS
  Edge Detector2 : dspswit3/Edge Detector  InputProcessing=Columns as channels (frame based)
      settings: SourceProductName=DSP System Toolbox  SourceProductBaseCode=DS
  Gain : Gain  Gain=(2*pi)/500
  Gain4 : Gain  Gain=1/2
  NOT : Logic  Operator=NOT  IconShape=distinctive  AllPortsSameDT=off  OutDataTypeStr=boolean
  OR : Logic  Operator=OR  IconShape=distinctive  AllPortsSameDT=off  OutDataTypeStr=boolean
  Periode : Product  Inputs=*/
  Periode meting : MATLAB Function  TreatAsAtomicUnit=on
  Out : Outport
  wires:
  Constant3/1 -> Periode/2, Periode meting/2(period)
  Periode/1 -> Gain/1, Display4/1
  Constant2/1 -> Periode meting/3(fs)
  Periode meting/1(pulses) -> Periode/1
  In/1 -> NOT/1, Edge Detector1/1
  Gain/1 -> Gain4/1
  OR/1 -> Periode meting/1(speedPulse)
  Edge Detector1/1 -> OR/1
  Edge Detector2/1 -> OR/2
  NOT/1 -> Edge Detector2/1
  Gain4/1 -> Out/1
  Constant/1 -> Periode meting/4(reset)

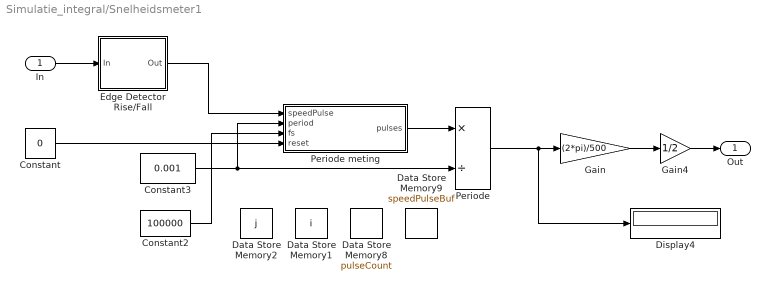
== system Simulatie_integral/Snelheidsmeter1 ==
  In : Inport
  Constant : Constant  Value=0
  Constant2 : Constant  Value=100000
  Constant3 : Constant  Value=0.001
  Data Store Memory1 : DataStoreMemory  DataStoreName=i  ReadBeforeWriteMsg=warning  WriteAfterWriteMsg=warning  WriteAfterReadMsg=warning  InitialValue=1  ShowAdditionalParam=off  OutDataTypeStr=uint32
  Data Store Memory2 : DataStoreMemory  DataStoreName=j  ReadBeforeWriteMsg=warning  WriteAfterWriteMsg=warning  WriteAfterReadMsg=warning  InitialValue=2  ShowAdditionalParam=off  OutDataTypeStr=uint32
  Data Store Memory8 : DataStoreMemory  DataStoreName=pulseCount  ReadBeforeWriteMsg=warning  WriteAfterWriteMsg=warning  WriteAfterReadMsg=warning  ShowAdditionalParam=off  OutDataTypeStr=uint32
  Data Store Memory9 : DataStoreMemory  DataStoreName=speedPulseBuf  ReadBeforeWriteMsg=warning  WriteAfterWriteMsg=warning  WriteAfterReadMsg=warning  ShowAdditionalParam=off  OutDataTypeStr=uint8  Dimensions=10001
  Display4 : Display
  Edge Detector Rise/Fall : Subsystem
  Gain : Gain  Gain=(2*pi)/500
  Gain4 : Gain  Gain=1/2
  Periode : Product  Inputs=*/
  Periode meting : MATLAB Function  TreatAsAtomicUnit=on
  Out : Outport
  wires:
  Constant3/1 -> Periode/2, Periode meting/2(period)
  Periode/1 -> Gain/1, Display4/1
  Constant2/1 -> Periode meting/3(fs)
  Periode meting/1(pulses) -> Periode/1
  Gain/1 -> Gain4/1
  Constant/1 -> Periode meting/4(reset)
  Gain4/1 -> Out/1
  In/1 -> Edge Detector Rise/Fall/1(In)
  Edge Detector Rise/Fall/1(Out) -> Periode meting/1(speedPulse)

== system Simulatie_integral/Stroom links ==
  Demux : Demux  Tag=STV Demux  Outputs=1
  FromWs : FromWorkspace  Tag=STV FromWs  VariableName=tuvar  SampleTime=0
      SigBuilderData=|
      | common.afterFinalStr = 'Extrapolate'
      | common.sampleTime = 0
      | dataSet.timeRange = [0 10]
      | dataSet.name = 'Group 1'
      | sbobj.Groups.Name = 'Group 1'
      | sbobj.Groups.Signals.Name = 'Signal 1'
      | sbobj.Groups.Signals.XData = [0 1 1.5 2 7 10]
      | sbobj.Groups.Signals.YData = [0 0 30 0 0 0]
  Signal 1 : Outport  Tag=STV Outport
  wires:
  Demux/1 -> Signal 1/1
  FromWs/1 -> Demux/1

== system Simulatie_integral/Stroom rechts ==
  Demux : Demux  Tag=STV Demux  Outputs=1
  FromWs : FromWorkspace  Tag=STV FromWs  VariableName=tuvar  SampleTime=0
      SigBuilderData=|
      | common.afterFinalStr = 'Extrapolate'
      | common.sampleTime = 0
      | dataSet.timeRange = [0 10]
      | dataSet.name = 'Group 1'
      | sbobj.Groups.Name = 'Group 1'
      | sbobj.Groups.Signals.Name = 'Signal 1'
      | sbobj.Groups.Signals.XData = [0 1 1.5 2 7 10]
      | sbobj.Groups.Signals.YData = [0 0 30 0 0 0]
  Signal 1 : Outport  Tag=STV Outport
  wires:
  Demux/1 -> Signal 1/1
  FromWs/1 -> Demux/1

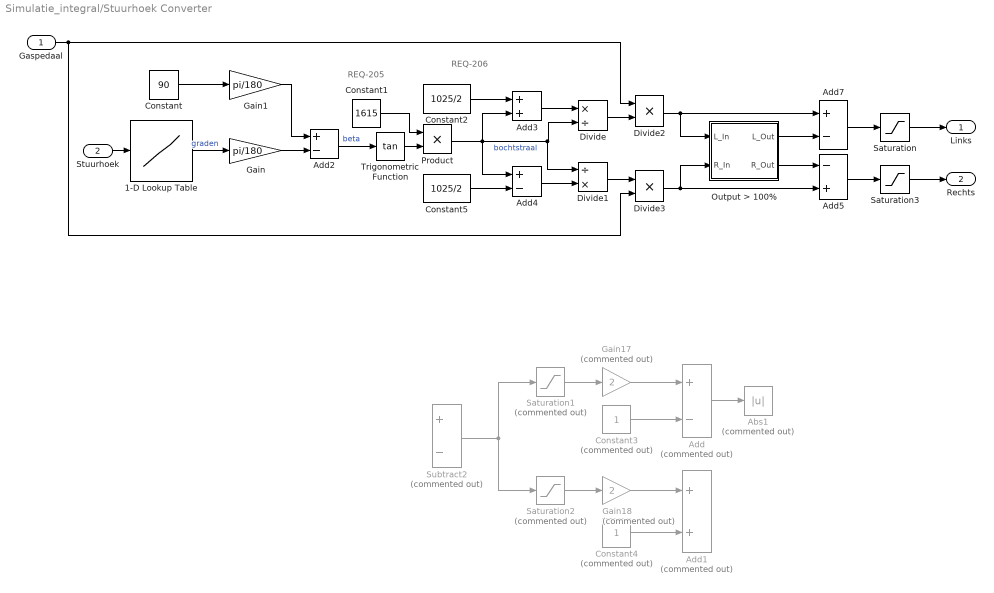
== system Simulatie_integral/Stuurhoek Converter ==
  note: REQ-205
  note: REQ-206
  "Gaspedaal " : Inport
  Stuurhoek : Inport  Port=2
  1-D Lookup Table : Lookup_n-D  NumberOfTableDimensions=1  BreakpointsForDimension1=[0 0.5 1]  Table=[-30 0 30]  InternalRulePriority=Speed  RndMeth=Simplest  InputSameDT=on
  Abs1 : Abs  Commented=on
  Add : Sum  Commented=on  Inputs=+-
  Add1 : Sum  Commented=on
  Add2 : Sum  Inputs=+-
  Add3 : Sum
  Add4 : Sum  Inputs=+-
  Add5 : Sum  Inputs=-+
  Add7 : Sum  Inputs=+-
  Constant : Constant  Value=90
  Constant1 : Constant  Value=1615
  Constant2 : Constant  Value=1025/2
  Constant3 : Constant  Commented=on
  Constant4 : Constant  Commented=on
  Constant5 : Constant  Value=1025/2
  Divide : Product  Inputs=*/
  Divide1 : Product  Inputs=/*
  Divide2 : Product  Inputs=**
  Divide3 : Product  Inputs=**
  Gain : Gain  Gain=pi/180
  Gain1 : Gain  Gain=pi/180
  Gain17 : Gain  Commented=on  Gain=2
  Gain18 : Gain  Commented=on  Gain=2
  Output > 100% : Subsystem
  Product : Product
  Saturation : Saturate  UpperLimit=1  LowerLimit=0
  Saturation1 : Saturate  Commented=on  LowerLimit=0
  Saturation2 : Saturate  Commented=on  UpperLimit=0
  Saturation3 : Saturate  UpperLimit=1  LowerLimit=0
  Subtract2 : Sum  Commented=on  Inputs=+-
  Trigonometric Function : Trigonometry  Operator=tan
  Links : Outport
  Rechts : Outport  Port=2
  wires:
  Saturation1/1 -> Gain17/1
  Subtract2/1 -> Saturation2/1, Saturation1/1
  Gain18/1 -> Add1/1
  Add/1 -> Abs1/1
  Saturation2/1 -> Gain18/1
  Gain17/1 -> Add/1
  Constant4/1 -> Add1/2
  Constant3/1 -> Add/2
  1-D Lookup Table/1 -> Gain/1  "graden"
  Constant/1 -> Gain1/1
  Add2/1 -> Trigonometric Function/1  "beta"
  Constant1/1 -> Product/1
  Trigonometric Function/1 -> Product/2
  Product/1 -> Divide1/1, Divide/2, Add4/1, Add3/2  "bochtstraal"
  Constant2/1 -> Add3/1
  Add3/1 -> Divide/1
  Constant5/1 -> Add4/2
  Add4/1 -> Divide1/2
  Divide1/1 -> Divide3/1
  Divide/1 -> Divide2/2
  "Gaspedaal "/1 -> Divide2/1, Divide3/2
  Divide2/1 -> Add7/1, Output > 100%/1(L_In)
  Divide3/1 -> Output > 100%/2(R_In), Add5/2
  Stuurhoek/1 -> 1-D Lookup Table/1
  Gain/1 -> Add2/2
  Gain1/1 -> Add2/1
  Add7/1 -> Saturation/1
  Add5/1 -> Saturation3/1
  Output > 100%/1(L_Out) -> Add7/2
  Output > 100%/2(R_Out) -> Add5/1
  Saturation/1 -> Links/1
  Saturation3/1 -> Rechts/1

== system Simulatie_integral/Wisselend Input signal ==
  Demux : Demux  Tag=STV Demux  Outputs=1
  FromWs : FromWorkspace  Tag=STV FromWs  VariableName=tuvar  SampleTime=0
      SigBuilderData=|
      | common.afterFinalStr = 'Extrapolate'
      | common.sampleTime = 0
      | dataSet.timeRange = [0 10]
      | dataSet.name = 'Group 1'
      | sbobj.Groups.Name = 'Group 1'
      | sbobj.Groups.Signals.Name = 'Signal 1'
      | sbobj.Groups.Signals.XData = [0 0.56 1 1 2 2 3 3 4 4 10]
      | sbobj.Groups.Signals.YData = [0 4 0 3.3 3.3 1 0 3.3 3.3 0 5]
  Signal 1 : Outport  Tag=STV Outport
  wires:
  Demux/1 -> Signal 1/1
  FromWs/1 -> Demux/1

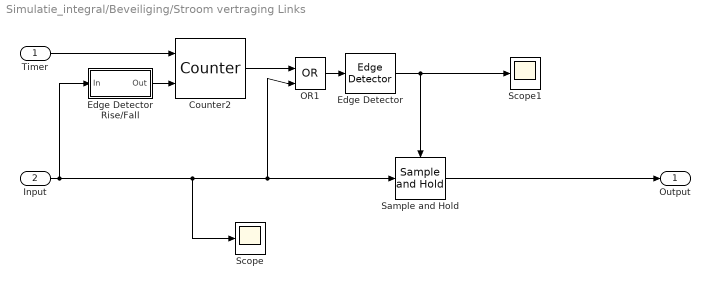
== system Simulatie_integral/Beveiliging/Stroom vertraging Links ==
  Timer : Inport
  Input : Inport  Port=2
  Counter2 : dspswit3/Counter  Direction=Up  CountEvent=Rising edge  CounterSize=User defined  MaxCount=300  InitialCount=0  Output=Hit  HitValue=300  ResetInput=on  SamplesPerFrame=1  Ts=1  CntDtype=double  HitDtype=Logical
  Edge Detector : dspswit3/Edge Detector  InputProcessing=Columns as channels (frame based)
      settings: SourceProductName=DSP System Toolbox  SourceProductBaseCode=DS
  Edge Detector Rise/Fall : Subsystem
  OR1 : Logic  Operator=OR  IconShape=distinctive  AllPortsSameDT=off  OutDataTypeStr=boolean
  Sample and Hold : dspsigops/Sample and Hold  trig=Rising edge  initCond=0  latchinput=off
  Scope : Scope
  Scope1 : Scope
  Output : Outport
  wires:
  Timer/1 -> Counter2/1
  Sample and Hold/1 -> Output/1
  OR1/1 -> Edge Detector/1
  Edge Detector/1 -> Scope1/1, Sample and Hold/Trigger
  Counter2/1 -> OR1/1
  Input/1 -> Scope/1, OR1/2, Sample and Hold/1, Edge Detector Rise/Fall/1(In)
  Edge Detector Rise/Fall/1(Out) -> Counter2/2

== system Simulatie_integral/Beveiliging/Stroom vertraging Rechts ==
  Timer : Inport
  Input : Inport  Port=2
  Counter2 : dspswit3/Counter  Direction=Up  CountEvent=Rising edge  CounterSize=User defined  MaxCount=300  InitialCount=0  Output=Hit  HitValue=300  ResetInput=on  SamplesPerFrame=1  Ts=1  CntDtype=double  HitDtype=Logical
  Edge Detector : dspswit3/Edge Detector  InputProcessing=Columns as channels (frame based)
      settings: SourceProductName=DSP System Toolbox  SourceProductBaseCode=DS
  Edge Detector Rise/Fall : Subsystem
  OR1 : Logic  Operator=OR  IconShape=distinctive  AllPortsSameDT=off  OutDataTypeStr=boolean
  Sample and Hold : dspsigops/Sample and Hold  trig=Rising edge  initCond=0  latchinput=off
  Scope : Scope
  Scope1 : Scope
  Output : Outport
  wires:
  Timer/1 -> Counter2/1
  Sample and Hold/1 -> Output/1
  OR1/1 -> Edge Detector/1
  Edge Detector/1 -> Scope1/1, Sample and Hold/Trigger
  Counter2/1 -> OR1/1
  Input/1 -> Scope/1, OR1/2, Sample and Hold/1, Edge Detector Rise/Fall/1(In)
  Edge Detector Rise/Fall/1(Out) -> Counter2/2

== system Simulatie_integral/Beveiliging/Temperatuur vertraging Links ==
  Timer : Inport
  Input : Inport  Port=2
  Counter2 : dspswit3/Counter  Direction=Up  CountEvent=Rising edge  CounterSize=User defined  MaxCount=300  InitialCount=0  Output=Hit  HitValue=300  ResetInput=on  SamplesPerFrame=1  Ts=1  CntDtype=double  HitDtype=Logical
  Edge Detector : dspswit3/Edge Detector  InputProcessing=Columns as channels (frame based)
      settings: SourceProductName=DSP System Toolbox  SourceProductBaseCode=DS
  Edge Detector Rise/Fall : Subsystem
  OR1 : Logic  Operator=OR  IconShape=distinctive  AllPortsSameDT=off  OutDataTypeStr=boolean
  Sample and Hold : dspsigops/Sample and Hold  trig=Rising edge  initCond=0  latchinput=off
  Scope : Scope
  Scope1 : Scope
  Output : Outport
  wires:
  Timer/1 -> Counter2/1
  Sample and Hold/1 -> Output/1
  OR1/1 -> Edge Detector/1
  Edge Detector/1 -> Scope1/1, Sample and Hold/Trigger
  Counter2/1 -> OR1/1
  Input/1 -> Scope/1, OR1/2, Sample and Hold/1, Edge Detector Rise/Fall/1(In)
  Edge Detector Rise/Fall/1(Out) -> Counter2/2

== system Simulatie_integral/Beveiliging/Temperatuur vertraging Rechts  ==
  Timer : Inport
  Input : Inport  Port=2
  Counter2 : dspswit3/Counter  Direction=Up  CountEvent=Rising edge  CounterSize=User defined  MaxCount=300  InitialCount=0  Output=Hit  HitValue=300  ResetInput=on  SamplesPerFrame=1  Ts=1  CntDtype=double  HitDtype=Logical
  Edge Detector : dspswit3/Edge Detector  InputProcessing=Columns as channels (frame based)
      settings: SourceProductName=DSP System Toolbox  SourceProductBaseCode=DS
  Edge Detector Rise/Fall : Subsystem
  OR1 : Logic  Operator=OR  IconShape=distinctive  AllPortsSameDT=off  OutDataTypeStr=boolean
  Sample and Hold : dspsigops/Sample and Hold  trig=Rising edge  initCond=0  latchinput=off
  Scope : Scope
  Scope1 : Scope
  Output : Outport
  wires:
  Timer/1 -> Counter2/1
  Sample and Hold/1 -> Output/1
  OR1/1 -> Edge Detector/1
  Edge Detector/1 -> Scope1/1, Sample and Hold/Trigger
  Counter2/1 -> OR1/1
  Input/1 -> Scope/1, OR1/2, Sample and Hold/1, Edge Detector Rise/Fall/1(In)
  Edge Detector Rise/Fall/1(Out) -> Counter2/2

== system Simulatie_integral/Snelheidsmeter1/Edge Detector Rise//Fall ==
  In : Inport
  Edge Detector1 : dspswit3/Edge Detector  InputProcessing=Columns as channels (frame based)
      settings: SourceProductName=DSP System Toolbox  SourceProductBaseCode=DS
  Edge Detector2 : dspswit3/Edge Detector  InputProcessing=Columns as channels (frame based)
      settings: SourceProductName=DSP System Toolbox  SourceProductBaseCode=DS
  NOT : Logic  Operator=NOT  IconShape=distinctive  AllPortsSameDT=off  OutDataTypeStr=boolean
  OR : Logic  Operator=OR  IconShape=distinctive  AllPortsSameDT=off  OutDataTypeStr=boolean
  Out : Outport
  wires:
  In/1 -> NOT/1, Edge Detector1/1
  NOT/1 -> Edge Detector2/1
  Edge Detector1/1 -> OR/1
  OR/1 -> Out/1
  Edge Detector2/1 -> OR/2

== system Simulatie_integral/Stuurhoek Converter/Output > 100% ==
  L_In : Inport
  R_In : Inport  Port=2
  Compare To Constant : simulink/Logic and Bit Operations/Compare To Constant  relop=>  const=1  OutDataTypeStr=boolean
  Compare To Constant1 : simulink/Logic and Bit Operations/Compare To Constant  relop=>  const=1  OutDataTypeStr=boolean
  Divide4 : Product  Inputs=**
  Divide5 : Product  Inputs=**
  Subtract : Sum  Inputs=+-
  Subtract1 : Sum  Inputs=-+
  L_Out : Outport
  R_Out : Outport  Port=2
  wires:
  Compare To Constant1/1 -> Subtract1/1, Divide4/1
  Compare To Constant/1 -> Subtract/2, Divide5/2
  Subtract1/1 -> Divide4/2
  Subtract/1 -> Divide5/1
  L_In/1 -> Subtract/1, Compare To Constant/1
  Divide5/1 -> R_Out/1
  R_In/1 -> Subtract1/2, Compare To Constant1/1
  Divide4/1 -> L_Out/1

== system Simulatie_integral/Beveiliging/Stroom vertraging Links/Edge Detector Rise//Fall ==
  In : Inport
  Edge Detector1 : dspswit3/Edge Detector  InputProcessing=Columns as channels (frame based)
      settings: SourceProductName=DSP System Toolbox  SourceProductBaseCode=DS
  Edge Detector2 : dspswit3/Edge Detector  InputProcessing=Columns as channels (frame based)
      settings: SourceProductName=DSP System Toolbox  SourceProductBaseCode=DS
  NOT : Logic  Operator=NOT  IconShape=distinctive  AllPortsSameDT=off  OutDataTypeStr=boolean
  OR : Logic  Operator=OR  IconShape=distinctive  AllPortsSameDT=off  OutDataTypeStr=boolean
  Out : Outport
  wires:
  In/1 -> NOT/1, Edge Detector1/1
  NOT/1 -> Edge Detector2/1
  Edge Detector1/1 -> OR/1
  OR/1 -> Out/1
  Edge Detector2/1 -> OR/2

== system Simulatie_integral/Beveiliging/Stroom vertraging Rechts/Edge Detector Rise//Fall ==
  In : Inport
  Edge Detector1 : dspswit3/Edge Detector  InputProcessing=Columns as channels (frame based)
      settings: SourceProductName=DSP System Toolbox  SourceProductBaseCode=DS
  Edge Detector2 : dspswit3/Edge Detector  InputProcessing=Columns as channels (frame based)
      settings: SourceProductName=DSP System Toolbox  SourceProductBaseCode=DS
  NOT : Logic  Operator=NOT  IconShape=distinctive  AllPortsSameDT=off  OutDataTypeStr=boolean
  OR : Logic  Operator=OR  IconShape=distinctive  AllPortsSameDT=off  OutDataTypeStr=boolean
  Out : Outport
  wires:
  In/1 -> NOT/1, Edge Detector1/1
  NOT/1 -> Edge Detector2/1
  Edge Detector1/1 -> OR/1
  OR/1 -> Out/1
  Edge Detector2/1 -> OR/2

== system Simulatie_integral/Beveiliging/Temperatuur vertraging Links/Edge Detector Rise//Fall ==
  In : Inport
  Edge Detector1 : dspswit3/Edge Detector  InputProcessing=Columns as channels (frame based)
      settings: SourceProductName=DSP System Toolbox  SourceProductBaseCode=DS
  Edge Detector2 : dspswit3/Edge Detector  InputProcessing=Columns as channels (frame based)
      settings: SourceProductName=DSP System Toolbox  SourceProductBaseCode=DS
  NOT : Logic  Operator=NOT  IconShape=distinctive  AllPortsSameDT=off  OutDataTypeStr=boolean
  OR : Logic  Operator=OR  IconShape=distinctive  AllPortsSameDT=off  OutDataTypeStr=boolean
  Out : Outport
  wires:
  In/1 -> NOT/1, Edge Detector1/1
  NOT/1 -> Edge Detector2/1
  Edge Detector1/1 -> OR/1
  OR/1 -> Out/1
  Edge Detector2/1 -> OR/2

== system Simulatie_integral/Beveiliging/Temperatuur vertraging Rechts /Edge Detector Rise//Fall ==
  In : Inport
  Edge Detector1 : dspswit3/Edge Detector  InputProcessing=Columns as channels (frame based)
      settings: SourceProductName=DSP System Toolbox  SourceProductBaseCode=DS
  Edge Detector2 : dspswit3/Edge Detector  InputProcessing=Columns as channels (frame based)
      settings: SourceProductName=DSP System Toolbox  SourceProductBaseCode=DS
  NOT : Logic  Operator=NOT  IconShape=distinctive  AllPortsSameDT=off  OutDataTypeStr=boolean
  OR : Logic  Operator=OR  IconShape=distinctive  AllPortsSameDT=off  OutDataTypeStr=boolean
  Out : Outport
  wires:
  In/1 -> NOT/1, Edge Detector1/1
  NOT/1 -> Edge Detector2/1
  Edge Detector1/1 -> OR/1
  OR/1 -> Out/1
  Edge Detector2/1 -> OR/2

== matlab function Simulatie_integral/Snelheidsmeter1/Periode meting ==
  data: speedPulse input; pulses output; speedPulseBuf data_store_memory; pulseCount data_store_memory; period input; i data_store_memory; fs input; j data_store_memory; reset input
function pulses = fcn(speedPulse,period, fs, reset)

global pulseCount;
global speedPulseBuf;
global i;
global j;

if reset == 1
    speedPulseBuf = uint8(zeros(size(speedPulseBuf)));
end

bufTime = period*fs + 1;

if i > bufTime
    i = uint32(1);
end

if j > bufTime
    j = uint32(1);
end

speedPulseBuf(i) = speedPulse;
pulseCount = pulseCount + uint32(speedPulse);
pulseCount = pulseCount - uint32(speedPulseBuf(j));

i = i + 1;
j = j + 1;

pulses = pulseCount;

== matlab function Simulatie_integral/Snelheidsmeter/Periode meting ==
  data: speedPulse input; pulses output; speedPulseBuf data_store_memory; pulseCount data_store_memory; period input; i data_store_memory; fs input; j data_store_memory; reset input
function pulses = fcn(speedPulse,period, fs, reset)

global pulseCount;
global speedPulseBuf;
global i;
global j;

if reset == 1
    speedPulseBuf = uint8(zeros(size(speedPulseBuf)));
end

bufTime = period*fs + 1;

if i > bufTime
    i = uint32(1);
end

if j > bufTime
    j = uint32(1);
end

speedPulseBuf(i) = speedPulse;
pulseCount = pulseCount + uint32(speedPulse);
pulseCount = pulseCount - uint32(speedPulseBuf(j));

i = i + 1;
j = j + 1;

pulses = pulseCount;
